simulink model "ALU1Bit"  (R2023a)
settings: Solver=VariableStepAuto  StartTime=0.0  StopTime=1  RelTol=1e-3
settings Model: Creator=Admin  LastModifiedBy=Admin

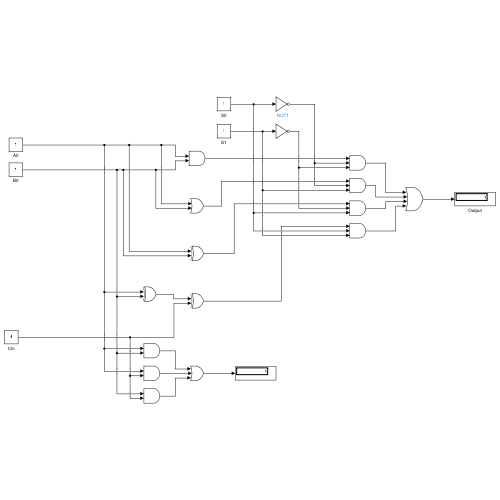
[thumbnail: Simulink's stored preview of the top-level diagram]
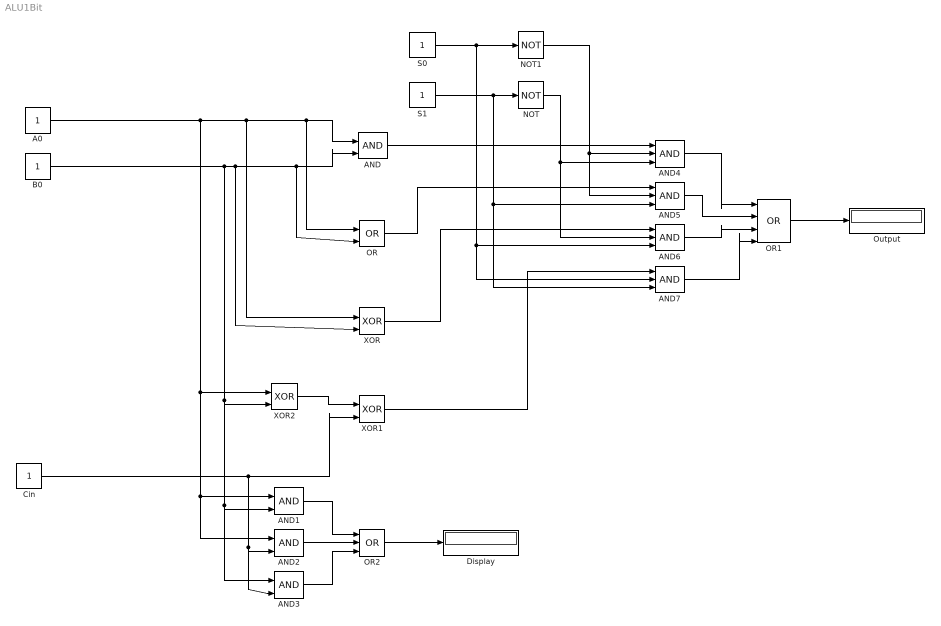
== system ALU1Bit ==
  A0 : Constant  SampleTime=-1
  AND{,1..3} (4 alike) : Logic  IconShape=distinctive  AllPortsSameDT=off  OutDataTypeStr=boolean
  AND{4..7} (4 alike) : Logic  Inputs=3  IconShape=distinctive  AllPortsSameDT=off  OutDataTypeStr=boolean
  B0 : Constant  SampleTime=-1
  Cin : Constant  SampleTime=-1
  Display : Display
  NOT : Logic  Operator=NOT  IconShape=distinctive  AllPortsSameDT=off  OutDataTypeStr=boolean
  NOT1 : Logic  Operator=NOT  IconShape=distinctive  AllPortsSameDT=off  OutDataTypeStr=boolean
  OR : Logic  Operator=OR  IconShape=distinctive  AllPortsSameDT=off  OutDataTypeStr=boolean
  OR1 : Logic  Operator=OR  Inputs=4  IconShape=distinctive  AllPortsSameDT=off  OutDataTypeStr=boolean
  OR2 : Logic  Operator=OR  Inputs=3  IconShape=distinctive  AllPortsSameDT=off  OutDataTypeStr=boolean
  Output : Display
  S0 : Constant  SampleTime=-1
  S1 : Constant  SampleTime=-1
  XOR : Logic  Operator=XOR  IconShape=distinctive  AllPortsSameDT=off  OutDataTypeStr=boolean
  XOR1 : Logic  Operator=XOR  IconShape=distinctive  AllPortsSameDT=off  OutDataTypeStr=boolean
  XOR2 : Logic  Operator=XOR  IconShape=distinctive  AllPortsSameDT=off  OutDataTypeStr=boolean
  wires:
  XOR2/1 -> XOR1/1
  A0/1 -> AND1/1, AND2/1, XOR2/1, XOR/1, OR/1, AND/1
  B0/1 -> AND1/2, AND3/1, XOR2/2, XOR/2, OR/2, AND/2
  Cin/1 -> AND2/2, AND3/2, XOR1/2
  S1/1 -> AND7/3, AND5/3, NOT/1
  S0/1 -> AND7/2, AND6/3, NOT1/1
  NOT1/1 -> AND4/2, AND5/2
  NOT/1 -> AND6/2, AND4/3
  AND/1 -> AND4/1
  OR/1 -> AND5/1
  XOR/1 -> AND6/1
  XOR1/1 -> AND7/1
  AND4/1 -> OR1/1
  AND5/1 -> OR1/2
  AND6/1 -> OR1/3
  AND7/1 -> OR1/4
  OR1/1 -> Output/1
  OR2/1 -> Display/1
  AND2/1 -> OR2/2
  AND1/1 -> OR2/1
  AND3/1 -> OR2/3
